simulink model "vloop_load"  (R2022b)
settings: Solver=ode15s  StartTime=0.0  StopTime=1.0  RelTol=1e-3  EnableMultiTasking=on
InitFcn:
  | G = 107.815;
undefined symbols (not defined in the file): InertiaA, R, torq_const, torq_max
libraries: roblocks x6, simulink x1
Description:
  | vloop parameters for
  | Puma560 shoulder joint
  | with link inertia
  | RVC1 p.205
settings Model: DisableUpgradeWarningsForVersion=R2014b  Creator=pic  LastModifiedBy=Artem
settings SolverCC: AlgebraicLoopSolver=TrustRegion
settings DataIOCC: LimitDataPoints=on  SaveFormat=Array  SignalLoggingSaveFormat=ModelDataLogs  TimeSaveName=t  OutputSaveName=y
settings OptimizationCC: ExpressionDepthLimit=2147483647  LifeSpan=inf
settings DebuggingCC: UnderspecifiedInitializationDetection=Classic  MergeDetectMultiDrivingBlocksExec=none  SolverPrmCheckMsg=warning  MultiTaskRateTransMsg=warning  FcnCallInpInsideContextMsg=warning  UnconnectedInputMsg=warning  UnconnectedOutputMsg=warning  UnconnectedLineMsg=warning  AllowSymbolicDim=off  StateNameClashWarn=warning  SFUnexpectedBacktrackingDiag=warning  SFNoUnconditionalDefaultTransitionDiag=warning  SFExecutionAtInitializationDiag=none  SFMachineParentedDataDiag=warning  ArithmeticOperatorsInVariantConditions=warning
settings HardwareCC: ProdBitPerPointer=32  ProdBitPerSizeT=32  ProdBitPerPtrDiffT=32  ProdLargestAtomicFloat=None  ProdIntDivRoundTo=Undefined  ProdEndianess=Unspecified  ProdWordSize=32  ProdHWDeviceType=32-bit Generic
settings ModelReferenceCC: EnableRefExpFcnMdlSchedulingChecks=on  PropagateSignalLabelsOutOfModel=off
settings SFSimCC: SimUseLocalCustomCode=off  CustomCodeUndefinedFunction=UseInterfaceOnly
settings SFSimCC: SimCustomInitializer=|
  | if ~exist(tau_d)
  |    tau_d = 0
  | end
settings RTWCC: RTWUseLocalCustomCode=off  DLArmComputeVersion=19.05
settings CodeAppCC: StateflowObjectComments=on
settings GRTTargetCC: TargetLangStandard=C89/C90 (ANSI)  CombineOutputUpdateFcns=off  GRTInterface=on
settings ConfigComp: CovMetricSettings=dw  CovSaveCumulativeToWorkspaceVar=on  CovSaveSingleToWorkspaceVar=on  CovExternalEMLEnable=off  CovSFcnEnable=off

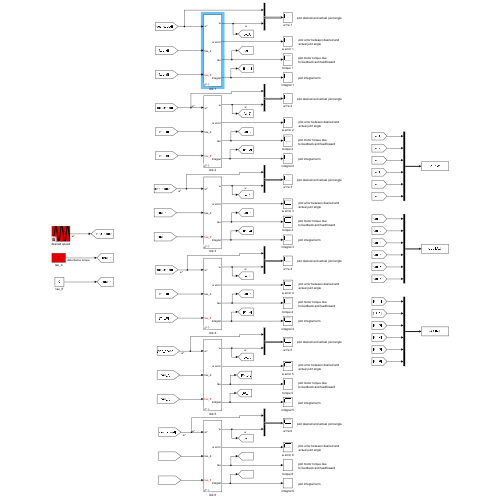
[thumbnail: Simulink's stored preview of the top-level diagram]
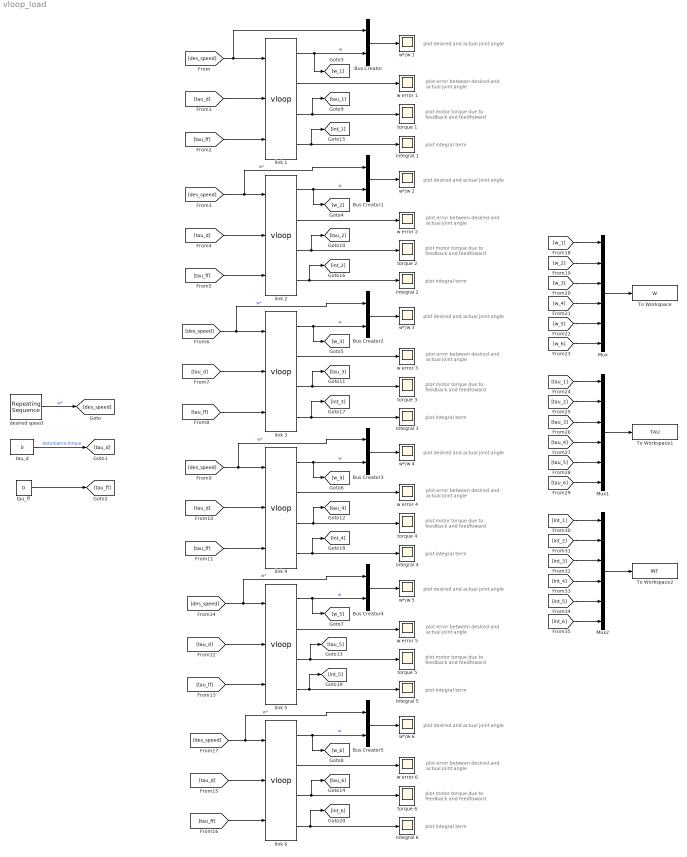
== system vloop_load ==
  note: plot integral term
  note: plot motor torque due
      | to feedback and feedfoward
  note: plot error between desired and
      | actual joint angle
  note: plot desired and actual joint angle
  note: plot integral term
  note: plot motor torque due
      | to feedback and feedfoward
  note: plot error between desired and
      | actual joint angle
  note: plot desired and actual joint angle
  note: plot integral term
  note: plot motor torque due
      | to feedback and feedfoward
  note: plot error between desired and
      | actual joint angle
  note: plot desired and actual joint angle
  note: plot integral term
  note: plot motor torque due
      | to feedback and feedfoward
  note: plot error between desired and
      | actual joint angle
  note: plot desired and actual joint angle
  note: plot integral term
  note: plot motor torque due
      | to feedback and feedfoward
  note: plot error between desired and
      | actual joint angle
  note: plot desired and actual joint angle
  note: plot integral term
  note: plot motor torque due
      | to feedback and feedfoward
  note: plot error between desired and
      | actual joint angle
  note: plot desired and actual joint angle
  Bus Creator{,1..5} (6 alike) : BusCreator  Inputs=2
  Mux : Mux  Inputs=6
  Mux1 : Mux  Inputs=6
  Mux2 : Mux  Inputs=6
  To Workspace : ToWorkspace  VariableName=W  SaveFormat=Timeseries  SampleTime=-1
  To Workspace1 : ToWorkspace  VariableName=TAU  SaveFormat=Timeseries  SampleTime=-1
  To Workspace2 : ToWorkspace  VariableName=INT  SaveFormat=Timeseries  SampleTime=-1
  desired speed : simulink/Sources/Repeating Sequence  rep_seq_t=[0 1 3 4 6]/10  rep_seq_y=[0 0 50 50 0]
  integral {1..6} (6 alike) : Scope
  link 1 : roblocks/Arm/vloop  J=InertiaA(1)  B=R.links(1,1).B  Km=torq_const(1)  tau_max=torq_max(1)  Kv=5  Ki=6  T=0.001
  link 2 : roblocks/Arm/vloop  J=InertiaA(2)  B=R.links(1,2).B  Km=torq_const(2)  tau_max=torq_max(2)  Kv=2.3  Ki=3  T=0.001
  link 3 : roblocks/Arm/vloop  J=InertiaA(3)  B=R.links(1,3).B  Km=torq_const(3)  tau_max=torq_max(3)  Kv=2.5  Ki=3  T=0.001
  link 4 : roblocks/Arm/vloop  J=InertiaA(4)  B=R.links(1,4).B  Km=torq_const(4)  tau_max=torq_max(4)  Kv=1.5  Ki=2  T=0.001
  link 5 : roblocks/Arm/vloop  J=InertiaA(5)  B=R.links(1,5).B  Km=torq_const(5)  tau_max=torq_max(5)  Kv=2  Ki=2  T=0.001
  link 6 : roblocks/Arm/vloop  J=InertiaA(6)  B=R.links(1,6).B  Km=torq_const(6)  tau_max=torq_max(6)  Kv=5  Ki=5  T=0.001
  tau_d : Constant  Value=0
  tau_ff : Constant  Value=0
  torque {1..6} (6 alike) : Scope
  w error {1..6} (6 alike) : Scope
  w*/w {1..6} (6 alike) : Scope
  wires:
  Bus Creator/1 -> w*/w 1/1
  link 1/1 -> [w_1], Bus Creator/2  "w"
  link 1/2 -> w error 1/1
  link 1/3 -> [tau_1], torque 1/1
  link 1/4 -> [int_1], integral 1/1
  link 2/4 -> [int_2], integral 2/1
  link 2/3 -> [tau_2], torque 2/1
  link 2/2 -> w error 2/1
  link 2/1 -> [w_2], Bus Creator1/2  "w"
  Bus Creator1/1 -> w*/w 2/1
  [des_speed] -> Bus Creator1/1, link 2/1  "w*"
  Bus Creator2/1 -> w*/w 3/1
  link 3/1 -> [w_3], Bus Creator2/2  "w"
  link 3/2 -> w error 3/1
  link 3/3 -> [tau_3], torque 3/1
  link 3/4 -> [int_3], integral 3/1
  link 4/4 -> [int_4], integral 4/1
  link 4/3 -> [tau_4], torque 4/1
  link 4/2 -> w error 4/1
  link 4/1 -> [w_4], Bus Creator3/2  "w"
  Bus Creator3/1 -> w*/w 4/1
  Bus Creator4/1 -> w*/w 5/1
  link 5/1 -> [w_5], Bus Creator4/2  "w"
  link 5/2 -> w error 5/1
  link 5/3 -> [tau_5], torque 5/1
  link 5/4 -> [int_5], integral 5/1
  link 6/4 -> [int_6], integral 6/1
  link 6/3 -> [tau_6], torque 6/1
  link 6/2 -> w error 6/1
  link 6/1 -> [w_6], Bus Creator5/2  "w"
  Bus Creator5/1 -> w*/w 6/1
  [des_speed] -> Bus Creator5/1, link 6/1  "w*"
  desired speed/1 -> [des_speed]  "w*"
  tau_d/1 -> [tau_d]  "disturbance torque"
  tau_ff/1 -> [tau_ff]
  [des_speed] -> Bus Creator/1, link 1/1
  [tau_d] -> link 1/2
  [tau_ff] -> link 1/3
  [tau_d] -> link 2/2
  [tau_ff] -> link 2/3
  [des_speed] -> Bus Creator2/1, link 3/1  "w*"
  [tau_d] -> link 3/2
  [tau_ff] -> link 3/3
  [des_speed] -> Bus Creator3/1, link 4/1  "w*"
  [tau_d] -> link 4/2
  [tau_ff] -> link 4/3
  [tau_ff] -> link 5/3
  [tau_d] -> link 5/2
  [des_speed] -> Bus Creator4/1, link 5/1  "w*"
  [tau_ff] -> link 6/3
  [tau_d] -> link 6/2
  [w_1] -> Mux/1
  [w_2] -> Mux/2
  [w_3] -> Mux/3
  [w_4] -> Mux/4
  [w_5] -> Mux/5
  [w_6] -> Mux/6
  Mux/1 -> To Workspace/1
  [tau_6] -> Mux1/6
  [tau_5] -> Mux1/5
  [tau_4] -> Mux1/4
  [tau_3] -> Mux1/3
  [tau_2] -> Mux1/2
  [tau_1] -> Mux1/1
  [int_1] -> Mux2/1
  [int_2] -> Mux2/2
  [int_3] -> Mux2/3
  [int_4] -> Mux2/4
  [int_5] -> Mux2/5
  [int_6] -> Mux2/6
  Mux1/1 -> To Workspace1/1
  Mux2/1 -> To Workspace2/1
